simulink model "Sim_CVBT"  (R2022a)
settings: Solver=ode45  StartTime=0.0  StopTime=600  FixedStep=0.01  RelTol=1e-3  EnableMultiTasking=on
InitFcn:
  | initialize;
  | %graphics_init;
values from neighbouring files (symbols this model uses):
  a = 0.08    [initialize.m]
  b = 0.002*0    (= 0)    [initialize.m]
  Kdv = 0    [initialize.m]
  Kiv = 0    [initialize.m]
  Kpsi = 2    [initialize.m]
  Kpv = 0.2    [initialize.m]
  numVeh = 6    [initialize.m]
  P0 = zeros(40,1)    [initialize.m]
  P0tg = [-400 -400 0]    [initialize.m]
  psi0 = zeros(20,1)    [initialize.m]
  rho_d = [100 150 100 150 100 150 100 150 100 150]    [initialize.m]
  Vg = zeros(10,1)    [initialize.m]
  Vmax = 60    [initialize.m]
  Vmin = 10    [initialize.m]
  z0 = zeros(20,1)    [initialize.m]
libraries: slpidlib x6, simulink x2
(part 1 of 2)
settings Model: Creator=cichell2  LastModifiedBy=vcichella
settings SolverCC: AlgebraicLoopSolver=TrustRegion
settings DataIOCC: LimitDataPoints=on  SaveFormat=Array  SignalLoggingSaveFormat=ModelDataLogs  ReturnWorkspaceOutputs=off
settings OptimizationCC: ExpressionDepthLimit=2147483647  LifeSpan=inf
settings DebuggingCC: UnderspecifiedInitializationDetection=Classic  MergeDetectMultiDrivingBlocksExec=none  SolverPrmCheckMsg=warning  FcnCallInpInsideContextMsg=warning  UnconnectedInputMsg=warning  UnconnectedOutputMsg=warning  UnconnectedLineMsg=warning  StateNameClashWarn=warning  SFUnexpectedBacktrackingDiag=warning  SFNoUnconditionalDefaultTransitionDiag=warning  SFExecutionAtInitializationDiag=none  SFMachineParentedDataDiag=warning  ArithmeticOperatorsInVariantConditions=warning
settings HardwareCC: ProdBitPerPointer=32  ProdBitPerSizeT=32  ProdBitPerPtrDiffT=32  ProdLargestAtomicFloat=None  ProdIntDivRoundTo=Undefined  ProdEndianess=Unspecified  ProdWordSize=32  ProdHWDeviceType=32-bit Generic
settings ModelReferenceCC: PropagateSignalLabelsOutOfModel=off
settings SFSimCC: SimUseLocalCustomCode=off  CustomCodeUndefinedFunction=UseInterfaceOnly
settings RTWCC: RTWUseLocalCustomCode=off
settings CodeAppCC: StateflowObjectComments=on
settings GRTTargetCC: TargetLangStandard=C89/C90 (ANSI)  CombineOutputUpdateFcns=off  GRTInterface=on
settings ConfigComp: CovMetricSettings=dw  CovSaveCumulativeToWorkspaceVar=on  CovSaveSingleToWorkspaceVar=on  CovExternalEMLEnable=off

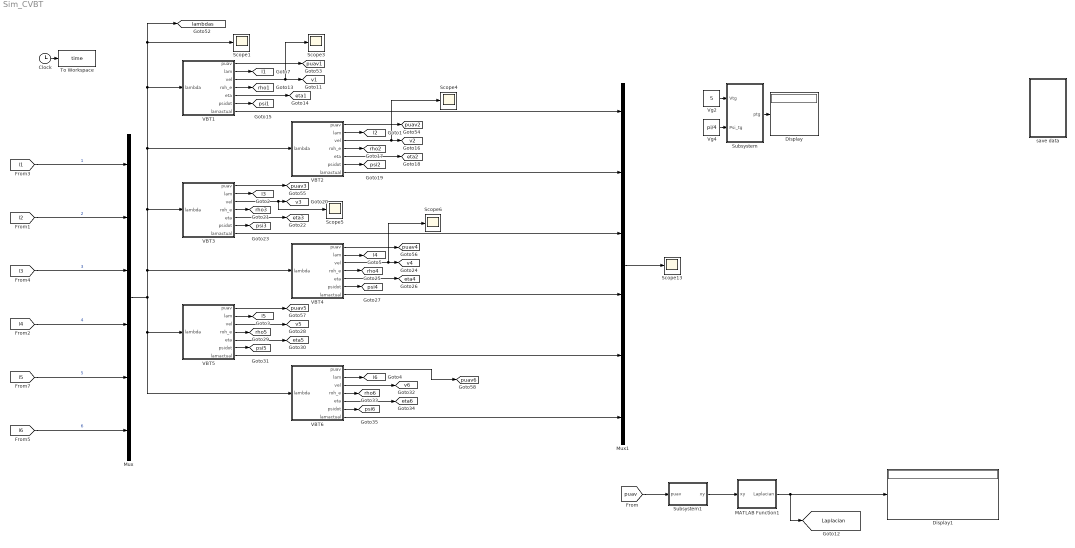
== system Sim_CVBT ==
  Clock : Clock
  Display : Display
  Display1 : Display
  MATLAB Function1 : MATLAB Function  TreatAsAtomicUnit=on
  Mux : Mux  Inputs=6
  Mux1 : Mux  Inputs=6
  Scope{1,3..6,13} (6 alike) : Scope
  Subsystem : Subsystem
  Subsystem1 : Subsystem
  To Workspace : ToWorkspace  VariableName=time  SampleTime=-1
  VBT1 : Subsystem  mask{UAV_no=1}
      mask prompts: UAV_no "UAV number"
  VBT2 : Subsystem  mask{UAV_no=2}
      mask prompts: UAV_no "UAV number"
  VBT3 : Subsystem  mask{UAV_no=3}
      mask prompts: UAV_no "UAV number"
  VBT4 : Subsystem  mask{UAV_no=4}
      mask prompts: UAV_no "UAV number"
  VBT5 : Subsystem  mask{UAV_no=5}
      mask prompts: UAV_no "UAV number"
  VBT6 : Subsystem  mask{UAV_no=6}
      mask prompts: UAV_no "UAV number"
  Vg2 : Constant  Value=5
  Vg4 : Constant  Value=pi/4
  save data : Subsystem
  tag scope: Laplacian=global, eta1=global, eta2=global, eta3=global, eta4=global, eta5=global, eta6=global, l1=global, l2=global, l3=global, l4=global, l5=global, l6=global, lambdas=global, psi1=global, psi2=global, psi3=global, psi4=global, psi5=global, psi6=global, puav1=global, puav2=global, puav3=global, puav4=global, puav5=global, puav6=global, rho1=global, rho2=global, rho3=global, rho4=global, rho5=global, rho6=global, v1=global, v2=global, v3=global, v4=global, v5=global, v6=global
  wires:
  Clock/1 -> To Workspace/1
  Vg2/1 -> Subsystem/1(Vtg)
  Vg4/1 -> Subsystem/2(Psi_tg)
  Subsystem/1(ptg) -> Display/1
  VBT1/2(lam) -> [l1]
  VBT2/2(lam) -> [l2]
  VBT3/2(lam) -> [l3]
  VBT5/2(lam) -> [l5]
  [l2] -> Mux/2  "2"
  [l1] -> Mux/1  "1"
  Mux/1 -> VBT5/1(lambda), VBT6/1(lambda), VBT3/1(lambda), [lambdas], Scope1/1, VBT1/1(lambda), VBT2/1(lambda), VBT4/1(lambda)
  [l4] -> Mux/4  "4"
  [l5] -> Mux/5  "5"
  [l6] -> Mux/6  "6"
  [l3] -> Mux/3  "3"
  VBT4/2(lam) -> [l4]
  VBT6/2(lam) -> [l6]
  VBT1/1(puav) -> [puav1]
  VBT2/1(puav) -> [puav2]
  VBT4/1(puav) -> [puav4]
  VBT5/1(puav) -> [puav5]
  VBT6/1(puav) -> [puav6]
  VBT1/3(vel) -> Scope3/1, [v1]
  VBT1/4(roh_e) -> [rho1]
  VBT1/5(eta) -> [eta1]
  VBT1/6(psidot) -> [psi1]
  VBT2/3(vel) -> Scope4/1, [v2]
  VBT2/5(eta) -> [eta2]
  VBT2/4(roh_e) -> [rho2]
  VBT2/6(psidot) -> [psi2]
  VBT3/3(vel) -> Scope5/1, [v3]
  VBT3/5(eta) -> [eta3]
  VBT3/4(roh_e) -> [rho3]
  VBT3/6(psidot) -> [psi3]
  VBT4/3(vel) -> Scope6/1, [v4]
  VBT4/5(eta) -> [eta4]
  VBT4/4(roh_e) -> [rho4]
  VBT4/6(psidot) -> [psi4]
  VBT5/3(vel) -> [v5]
  VBT5/5(eta) -> [eta5]
  VBT5/4(roh_e) -> [rho5]
  VBT5/6(psidot) -> [psi5]
  VBT6/3(vel) -> [v6]
  VBT6/5(eta) -> [eta6]
  VBT6/4(roh_e) -> [rho6]
  VBT6/6(psidot) -> [psi6]
  VBT3/1(puav) -> [puav3]
  [puav] -> Subsystem1/1(puav)
  MATLAB Function1/1(Laplacian) -> [Laplacian], Display1/1
  Subsystem1/1(xy) -> MATLAB Function1/1(xy)
  VBT1/7(lamactual) -> Mux1/1
  VBT2/7(lamactual) -> Mux1/2
  VBT3/7(lamactual) -> Mux1/3
  VBT4/7(lamactual) -> Mux1/4
  VBT5/7(lamactual) -> Mux1/5
  VBT6/7(lamactual) -> Mux1/6
  Mux1/1 -> Scope13/1

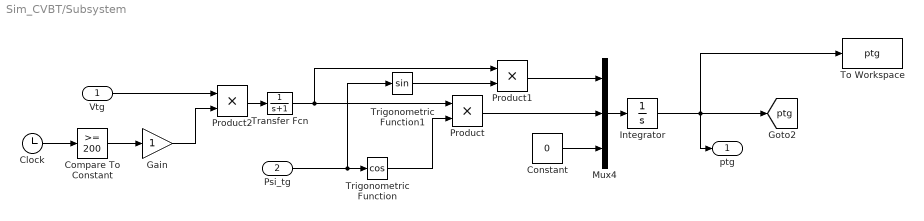
== system Sim_CVBT/Subsystem ==
  Vtg : Inport
  Psi_tg : Inport  Port=2
  Clock : Clock
  Compare To Constant : simulink/Logic and Bit Operations/Compare To Constant  relop=>=  const=200  OutDataTypeStr=boolean
  Constant : Constant  Value=0
  Gain : Gain
  Integrator : Integrator  InitialCondition=[P0tg(1) P0tg(2) P0tg(3)]  LimitOutput=on  UpperSaturationLimit=200  LowerSaturationLimit=-400
  Mux4 : Mux  Inputs=3
  Product : Product  RndMeth=Zero
  Product1 : Product  RndMeth=Zero
  Product2 : Product
  To Workspace : ToWorkspace  VariableName=ptg  SaveFormat=Timeseries  SampleTime=-1
  Transfer Fcn : TransferFcn  Denominator=[1 1]
  Trigonometric Function : Trigonometry  Operator=cos
  Trigonometric Function1 : Trigonometry
  ptg : Outport
  tag scope: ptg=global
  wires:
  Psi_tg/1 -> Trigonometric Function/1, Trigonometric Function1/1
  Integrator/1 -> To Workspace/1, ptg/1, [ptg]
  Mux4/1 -> Integrator/1
  Constant/1 -> Mux4/3
  Product/1 -> Mux4/2
  Trigonometric Function/1 -> Product/2
  Product1/1 -> Mux4/1
  Trigonometric Function1/1 -> Product1/2
  Clock/1 -> Compare To Constant/1
  Compare To Constant/1 -> Gain/1
  Product2/1 -> Transfer Fcn/1
  Vtg/1 -> Product2/1
  Gain/1 -> Product2/2
  Transfer Fcn/1 -> Product1/1, Product/1

== system Sim_CVBT/Subsystem1 ==
  puav : Inport
  Selector : Selector  InputPortWidth=18  IndexOptions=Index vector (dialog)  Indices=[1 2 4 5 7 8 10 11 13 14 16 17]  OutputSizes=1
  xy : Outport
  wires:
  puav/1 -> Selector/1
  Selector/1 -> xy/1

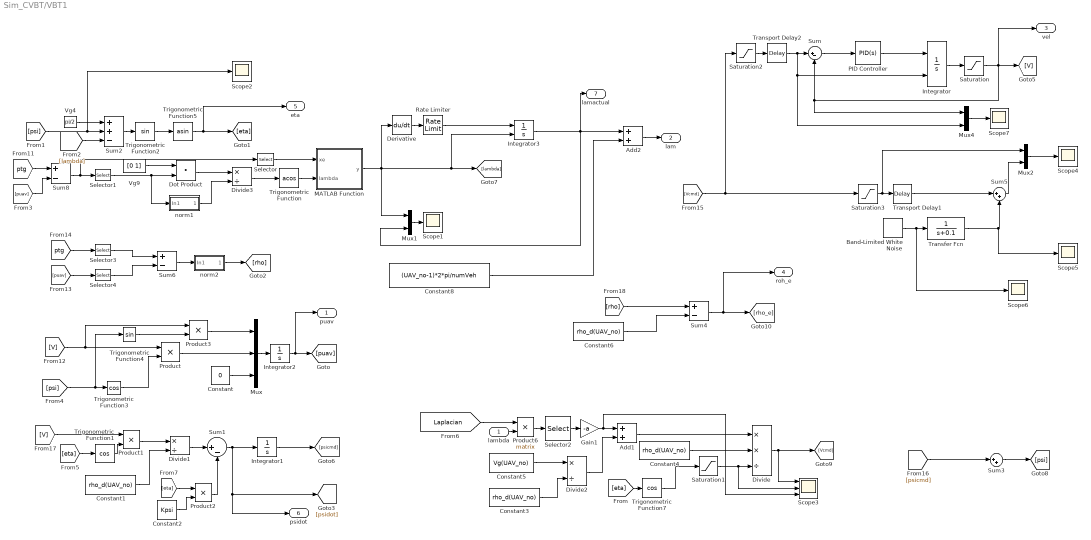
== system Sim_CVBT/VBT1 ==
  lambda : Inport
  Add1 : Sum
  Add2 : Sum
  Band-Limited White Noise : simulink/Sources/Band-Limited White Noise  Cov=[0.1]  Ts=0.1  seed=[23341]
  Constant : Constant  Value=0
  Constant{1,3..4,6} (4 alike) : Constant  Value=rho_d(UAV_no)
  Constant2 : Constant  Value=Kpsi
  Constant5 : Constant  Value=Vg(UAV_no)
  Constant8 : Constant  Value=(UAV_no-1)*2*pi/numVeh
  Derivative : Derivative
  Divide : Product  Inputs=**/
  Divide1 : Product  Inputs=*/
  Divide2 : Product  Inputs=*/
  Divide3 : Product  Inputs=*/
  Dot Product : DotProduct  OutDataTypeStr=Inherit: Inherit via internal rule
  Gain1 : Gain  Gain=-a
  Integrator : Integrator  InitialConditionSource=external
  Integrator1 : Integrator  InitialCondition=psi0(UAV_no)*pi/180
  Integrator2 : Integrator  InitialCondition=[P0(2*UAV_no-1) P0(2*UAV_no) z0(UAV_no)]
  Integrator3 : Integrator  InitialConditionSource=external
  MATLAB Function : MATLAB Function  TreatAsAtomicUnit=on
  Mux : Mux  Inputs=3
  Mux1 : Mux  Inputs=2
  Mux2 : Mux  Inputs=2
  Mux4 : Mux  Inputs=2
  PID Controller : slpidlib/PID Controller  Controller=PID  Form=Parallel  TimeDomain=Continuous-time  UseExternalTs=off  SampleTime=1  IntegratorMethod=Forward Euler  FilterMethod=Forward Euler  ControllerParametersSource=internal  P=Kpv  I=Kiv  UseKiTs=off  D=Kdv  N=100  UseFilter=on  TunerSelectOption=Transfer Function Based (PID Tuner App)  InitialConditionSource=internal  InitialConditionForIntegrator=0  InitialConditionForFilter=0  DifferentiatorICPrevScaledInput=0  ExternalReset=none  TrackingMode=off  Kt=1  LimitOutput=off  SatLimitsSource=internal  UpperSaturationLimit=inf  LowerSaturationLimit=-inf  LinearizeAsGain=on  AntiWindupMode=none  Kb=1  POutMin=[]  POutMax=[]  IOutMin=[]  IOutMax=[]  DOutMin=[]  DOutMax=[]  NOutMin=[]  NOutMax=[]  SumOutMin=[]  SumOutMax=[]  SaturationOutMin=[]  SaturationOutMax=[]  PParamMin=[]  PParamMax=[]  IParamMin=[]  IParamMax=[]  DParamMin=[]  DParamMax=[]  NParamMin=[]  NParamMax=[]  KbParamMin=[]  KbParamMax=[]  KtParamMin=[]  KtParamMax=[]  KbOutMin=[]  KbOutMax=[]  KtOutMin=[]  KtOutMax=[]  IntegratorOutMin=[]  IntegratorOutMax=[]  FilterOutMin=[]  FilterOutMax=[]  SumI1OutMin=[]  SumI1OutMax=[]  SumI2OutMin=[]  SumI2OutMax=[]  SumI3OutMin=[]  SumI3OutMax=[]  SumI4OutMin=[]  SumI4OutMax=[]  SumDOutMin=[]  SumDOutMax=[]  DifferentiatorOutMin=[]  DifferentiatorOutMax=[]  FilterDiffOutCoefMin=[]  FilterDiffOutCoefMax=[]  ReciprocalOutMin=[]  ReciprocalOutMax=[]  SumDenOutMin=[]  SumDenOutMax=[]  SumNumOutMin=[]  SumNumOutMax=[]  DivideOutMin=[]  DivideOutMax=[]  UdiffTsProdOutMin=[]  UdiffTsProdOutMax=[]  NTsProdOutMin=[]  NTsProdOutMax=[]  UintegralTsProdOutMin=[]  UintegralTsProdOutMax=[]  UngainTsProdOutMin=[]  UngainTsProdOutMax=[]  IntegratorContinuousStateAttributes=''  IntegratorStateMustResolveToSignalObject=off  IntegratorRTWStateStorageClass=Auto  FilterContinuousStateAttributes=''  FilterStateMustResolveToSignalObject=off  FilterRTWStateStorageClass=Auto  ParallelPVariant=InternalParameters  IdealPVariant=Disabled  IVariant=InternalParameters  DVariant=InternalParameters  IntegratorVariant=Continuous  SatVariant=Disabled  AWVariant=Passthrough  PCopyVariant=Disabled  TRVariant=Disabled  FdbkBlocksVariant=Forward  IdealPFdbkVariant=Disabled  SatFdbkVariant=Disabled  DerivativeFilterVariant=ContFilter  NVariant=InternalParameters  NCopyVariant=Disabled  FilterICVariant=InternalICsFilter  IntegratorICVariant=InternalICs  ExternalResetVariant=Disabled  TRSumVariant=Passthrough  SumFdbkVariant=Disabled  SumVariant=Sum_PID  TsampFilterVariant=InternalTs  TsampNgainVariant=Passthrough  TsampIntegralVariant=Passthrough  ExternalSaturationOutDataTypeStr=Inherit: Same as second input  aMode=0
  Product{,1..3} (4 alike) : Product  RndMeth=Zero
  Product6 : Product  Multiplication=Matrix(*)  RndMeth=Zero
  Rate Limiter : RateLimiter  RisingSlewLimit=100  FallingSlewLimit=-0.1  SampleTimeMode=inherited
  Saturation : Saturate  UpperLimit=Vmax  LowerLimit=Vmin
  Saturation1 : Saturate  UpperLimit=1  LowerLimit=0.8
  Saturation2 : Saturate  UpperLimit=Vmax  LowerLimit=Vmin
  Saturation3 : Saturate  UpperLimit=Vmax  LowerLimit=Vmin
  Scope{1..2,4..7} (6 alike) : Scope
  Scope3 : Scope  NumInputPorts=3
  Selector : Selector  InputPortWidth=3  IndexOptions=Index vector (dialog)  Indices=1  OutputSizes=1
  Selector1 : Selector  InputPortWidth=3  IndexOptions=Index vector (dialog)  Indices=[1 2]  OutputSizes=1
  Selector2 : Selector  InputPortWidth=6  IndexOptions=Index vector (dialog)  Indices=[UAV_no]  OutputSizes=1
  Selector3 : Selector  InputPortWidth=3  IndexOptions=Index vector (dialog)  Indices=[1 2]  OutputSizes=1
  Selector4 : Selector  InputPortWidth=3  IndexOptions=Index vector (dialog)  Indices=[1 2]  OutputSizes=1
  Sum : Sum  Inputs=|+-
  Sum1 : Sum  Inputs=|+-
  Sum2 : Sum  Inputs=++-
  Sum3 : Sum  Inputs=|++
  Sum4 : Sum  Inputs=+-
  Sum5 : Sum  Inputs=|++
  Sum6 : Sum  Inputs=+-
  Sum8 : Sum  Inputs=+-
  Transfer Fcn : TransferFcn  Denominator=[1 0.1]
  Transport Delay1 : TransportDelay  DelayTime=0.1
  Transport Delay2 : TransportDelay  DelayTime=0.1
  Trigonometric Function : Trigonometry  Operator=acos
  Trigonometric Function1 : Trigonometry  Operator=cos
  Trigonometric Function2 : Trigonometry
  Trigonometric Function3 : Trigonometry  Operator=cos
  Trigonometric Function4 : Trigonometry
  Trigonometric Function5 : Trigonometry  Operator=asin
  Trigonometric Function7 : Trigonometry  Operator=cos
  Vg4 : Constant  Value=pi/2
  Vg9 : Constant  Value=[0 1]
  norm1 : Subsystem
  norm2 : Subsystem
  puav : Outport
  lam : Outport  Port=2
  vel : Outport  Port=3
  roh_e : Outport  Port=4
  eta : Outport  Port=5
  psidot : Outport  Port=6
  lamactual : Outport  Port=7
  wires:
  Trigonometric Function1/1 -> Product1/2
  [eta] -> Trigonometric Function1/1
  Divide1/1 -> Sum1/1
  Product1/1 -> Divide1/1
  Constant1/1 -> Divide1/2
  [eta] -> Product2/1
  Product2/1 -> Sum1/2
  Constant2/1 -> Product2/2
  Sum1/1 -> Integrator1/1, psidot/1, [psidot]
  Sum6/1 -> norm2/1(In1)
  [puav] -> Selector4/1
  [ptg] -> Selector3/1
  Sum2/1 -> Trigonometric Function2/1
  Vg4/1 -> Sum2/1
  Sum8/1 -> Selector/1, Selector1/1
  [psi] -> Scope2/1, Sum2/2
  [lambda] -> Sum2/3
  Dot Product/1 -> Divide3/1
  norm1/1(Out1) -> Divide3/2
  [ptg] -> Sum8/1
  [puav] -> Sum8/2
  Integrator1/1 -> [psicmd]
  Selector/1 -> MATLAB Function/1(xe)
  Vg9/1 -> Dot Product/1
  Trigonometric Function2/1 -> Trigonometric Function5/1
  Trigonometric Function5/1 -> eta/1, [eta]
  [V] -> Product/1, Product3/1
  [psi] -> Trigonometric Function3/1, Trigonometric Function4/1
  Trigonometric Function3/1 -> Product/2
  Trigonometric Function4/1 -> Product3/2
  Product3/1 -> Mux/1
  Product/1 -> Mux/2
  Constant/1 -> Mux/3
  Mux/1 -> Integrator2/1
  Integrator2/1 -> puav/1, [puav]
  Selector1/1 -> Dot Product/2, norm1/1(In1)
  norm2/1(Out1) -> [rho]
  [V] -> Product1/1
  Mux1/1 -> Scope1/1
  [eta] -> Trigonometric Function7/1
  Add1/1 -> Divide/1
  Divide2/1 -> Add1/2
  Constant5/1 -> Divide2/1
  Constant3/1 -> Divide2/2
  Gain1/1 -> Scope3/3, Add1/1
  Trigonometric Function7/1 -> Saturation1/1
  Constant4/1 -> Divide/2
  Product6/1 -> Selector2/1
  [Laplacian] -> Product6/1
  lambda/1 -> Product6/2
  Selector2/1 -> Gain1/1
  Selector3/1 -> Sum6/1
  Selector4/1 -> Sum6/2
  Trigonometric Function/1 -> MATLAB Function/2(lambda)
  Divide3/1 -> Trigonometric Function/1
  MATLAB Function/1(y) -> Derivative/1, Mux1/1, Integrator3/2, [lambda]
  Derivative/1 -> Rate Limiter/1
  Integrator3/1 -> lamactual/1, Add2/1, Mux1/2
  Add2/1 -> lam/1
  Constant8/1 -> Add2/2
  Sum/1 -> PID Controller/1
  [psicmd] -> Sum3/1
  Sum3/1 -> [psi]
  [rho] -> Sum4/1
  Constant6/1 -> Sum4/2
  Sum4/1 -> roh_e/1, [rho_e]
  Saturation1/1 -> Scope3/2, Divide/3
  Saturation/1 -> [V], vel/1, Sum/2, Mux4/1
  Integrator/1 -> Saturation/1
  PID Controller/1 -> Integrator/1
  Mux4/1 -> Scope7/1
  Divide/1 -> Scope3/1, [Vcmd]
  Rate Limiter/1 -> Integrator3/1
  Saturation2/1 -> Transport Delay2/1
  [Vcmd] -> Saturation2/1, Saturation3/1
  Band-Limited White Noise/1 -> Scope6/1, Transfer Fcn/1
  Transfer Fcn/1 -> Scope5/1, Sum5/2
  Sum5/1 -> Mux2/2
  Mux2/1 -> Scope4/1
  Transport Delay1/1 -> Sum5/1
  Saturation3/1 -> Mux2/1, Transport Delay1/1
  Transport Delay2/1 -> Mux4/2, Integrator/2, Sum/1

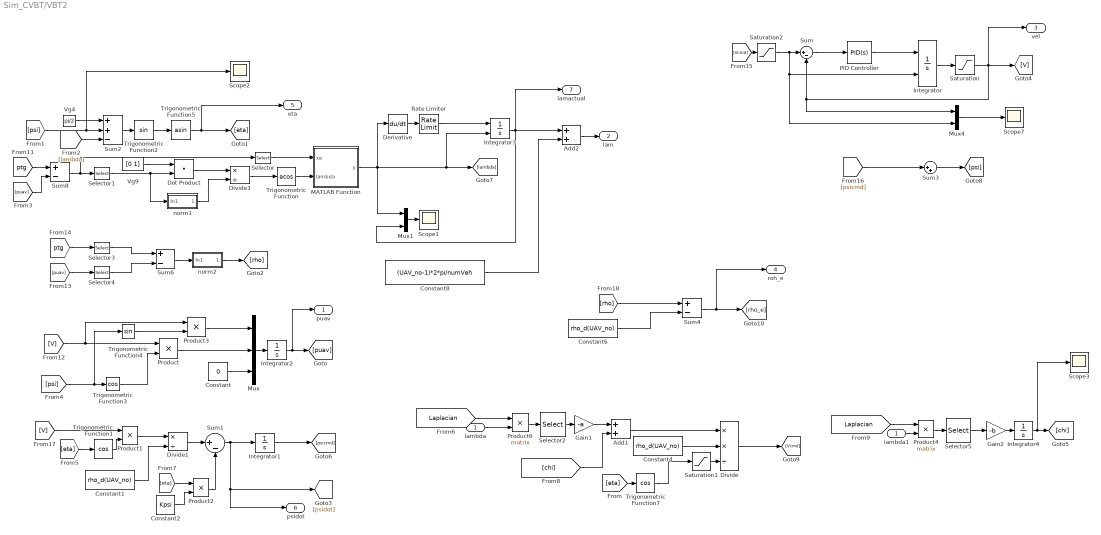
== system Sim_CVBT/VBT2 ==
  lambda : Inport
  Add1 : Sum
  Add2 : Sum
  Constant : Constant  Value=0
  Constant1 : Constant  Value=rho_d(UAV_no)
  Constant2 : Constant  Value=Kpsi
  Constant4 : Constant  Value=rho_d(UAV_no)
  Constant6 : Constant  Value=rho_d(UAV_no)
  Constant8 : Constant  Value=(UAV_no-1)*2*pi/numVeh
  Derivative : Derivative
  Divide : Product  Inputs=**/
  Divide1 : Product  Inputs=*/
  Divide3 : Product  Inputs=*/
  Dot Product : DotProduct  OutDataTypeStr=Inherit: Inherit via internal rule
  Gain1 : Gain  Gain=-a
  Gain2 : Gain  Gain=-b
  Integrator : Integrator  InitialConditionSource=external
  Integrator1 : Integrator  InitialCondition=psi0(UAV_no)*pi/180
  Integrator2 : Integrator  InitialCondition=[P0(2*UAV_no-1) P0(2*UAV_no) z0(UAV_no)]
  Integrator3 : Integrator  InitialConditionSource=external
  Integrator4 : Integrator  InitialCondition=Vg(UAV_no)/rho_d(UAV_no)
  MATLAB Function : MATLAB Function  TreatAsAtomicUnit=on
  Mux : Mux  Inputs=3
  Mux1 : Mux  Inputs=2
  Mux4 : Mux  Inputs=2
  PID Controller : slpidlib/PID Controller  Controller=PID  Form=Parallel  TimeDomain=Continuous-time  UseExternalTs=off  SampleTime=1  IntegratorMethod=Forward Euler  FilterMethod=Forward Euler  ControllerParametersSource=internal  P=Kpv  I=Kiv  UseKiTs=off  D=Kdv  N=100  UseFilter=on  TunerSelectOption=Transfer Function Based (PID Tuner App)  InitialConditionSource=internal  InitialConditionForIntegrator=0  InitialConditionForFilter=0  DifferentiatorICPrevScaledInput=0  ExternalReset=none  TrackingMode=off  Kt=1  LimitOutput=off  SatLimitsSource=internal  UpperSaturationLimit=inf  LowerSaturationLimit=-inf  LinearizeAsGain=on  AntiWindupMode=none  Kb=1  POutMin=[]  POutMax=[]  IOutMin=[]  IOutMax=[]  DOutMin=[]  DOutMax=[]  NOutMin=[]  NOutMax=[]  SumOutMin=[]  SumOutMax=[]  SaturationOutMin=[]  SaturationOutMax=[]  PParamMin=[]  PParamMax=[]  IParamMin=[]  IParamMax=[]  DParamMin=[]  DParamMax=[]  NParamMin=[]  NParamMax=[]  KbParamMin=[]  KbParamMax=[]  KtParamMin=[]  KtParamMax=[]  KbOutMin=[]  KbOutMax=[]  KtOutMin=[]  KtOutMax=[]  IntegratorOutMin=[]  IntegratorOutMax=[]  FilterOutMin=[]  FilterOutMax=[]  SumI1OutMin=[]  SumI1OutMax=[]  SumI2OutMin=[]  SumI2OutMax=[]  SumI3OutMin=[]  SumI3OutMax=[]  SumI4OutMin=[]  SumI4OutMax=[]  SumDOutMin=[]  SumDOutMax=[]  DifferentiatorOutMin=[]  DifferentiatorOutMax=[]  FilterDiffOutCoefMin=[]  FilterDiffOutCoefMax=[]  ReciprocalOutMin=[]  ReciprocalOutMax=[]  SumDenOutMin=[]  SumDenOutMax=[]  SumNumOutMin=[]  SumNumOutMax=[]  DivideOutMin=[]  DivideOutMax=[]  UdiffTsProdOutMin=[]  UdiffTsProdOutMax=[]  NTsProdOutMin=[]  NTsProdOutMax=[]  UintegralTsProdOutMin=[]  UintegralTsProdOutMax=[]  UngainTsProdOutMin=[]  UngainTsProdOutMax=[]  IntegratorContinuousStateAttributes=''  IntegratorStateMustResolveToSignalObject=off  IntegratorRTWStateStorageClass=Auto  FilterContinuousStateAttributes=''  FilterStateMustResolveToSignalObject=off  FilterRTWStateStorageClass=Auto  ParallelPVariant=InternalParameters  IdealPVariant=Disabled  IVariant=InternalParameters  DVariant=InternalParameters  IntegratorVariant=Continuous  SatVariant=Disabled  AWVariant=Passthrough  PCopyVariant=Disabled  TRVariant=Disabled  FdbkBlocksVariant=Forward  IdealPFdbkVariant=Disabled  SatFdbkVariant=Disabled  DerivativeFilterVariant=ContFilter  NVariant=InternalParameters  NCopyVariant=Disabled  FilterICVariant=InternalICsFilter  IntegratorICVariant=InternalICs  ExternalResetVariant=Disabled  TRSumVariant=Passthrough  SumFdbkVariant=Disabled  SumVariant=Sum_PID  TsampFilterVariant=InternalTs  TsampNgainVariant=Passthrough  TsampIntegralVariant=Passthrough  ExternalSaturationOutDataTypeStr=Inherit: Same as second input  aMode=0
  Product{,1..3} (4 alike) : Product  RndMeth=Zero
  Product4 : Product  Multiplication=Matrix(*)  RndMeth=Zero
  Product6 : Product  Multiplication=Matrix(*)  RndMeth=Zero
  Rate Limiter : RateLimiter  RisingSlewLimit=100  FallingSlewLimit=-0.1  SampleTimeMode=inherited
  Saturation : Saturate  UpperLimit=Vmax  LowerLimit=Vmin
  Saturation1 : Saturate  UpperLimit=1  LowerLimit=0.8
  Saturation2 : Saturate  UpperLimit=Vmax  LowerLimit=Vmin
  Scope{1..3,7} (4 alike) : Scope
  Selector : Selector  InputPortWidth=3  IndexOptions=Index vector (dialog)  Indices=1  OutputSizes=1
  Selector1 : Selector  InputPortWidth=3  IndexOptions=Index vector (dialog)  Indices=[1 2]  OutputSizes=1
  Selector2 : Selector  InputPortWidth=6  IndexOptions=Index vector (dialog)  Indices=[UAV_no]  OutputSizes=1
  Selector3 : Selector  InputPortWidth=3  IndexOptions=Index vector (dialog)  Indices=[1 2]  OutputSizes=1
  Selector4 : Selector  InputPortWidth=3  IndexOptions=Index vector (dialog)  Indices=[1 2]  OutputSizes=1
  Selector5 : Selector  InputPortWidth=6  IndexOptions=Index vector (dialog)  Indices=[UAV_no]  OutputSizes=1
  Sum : Sum  Inputs=|+-
  Sum1 : Sum  Inputs=|+-
  Sum2 : Sum  Inputs=++-
  Sum3 : Sum  Inputs=|++
  Sum4 : Sum  Inputs=+-
  Sum6 : Sum  Inputs=+-
  Sum8 : Sum  Inputs=+-
  Trigonometric Function : Trigonometry  Operator=acos
  Trigonometric Function1 : Trigonometry  Operator=cos
  Trigonometric Function2 : Trigonometry
  Trigonometric Function3 : Trigonometry  Operator=cos
  Trigonometric Function4 : Trigonometry
  Trigonometric Function5 : Trigonometry  Operator=asin
  Trigonometric Function7 : Trigonometry  Operator=cos
  Vg4 : Constant  Value=pi/2
  Vg9 : Constant  Value=[0 1]
  lambda1 : InportShadow
  norm1 : Subsystem
  norm2 : Subsystem
  puav : Outport
  lam : Outport  Port=2
  vel : Outport  Port=3
  roh_e : Outport  Port=4
  eta : Outport  Port=5
  psidot : Outport  Port=6
  lamactual : Outport  Port=7
  wires:
  Mux4/1 -> Scope7/1
  PID Controller/1 -> Integrator/1
  Integrator/1 -> Saturation/1
  Saturation/1 -> Mux4/1, Sum/2, [V], vel/1
  Saturation1/1 -> Divide/3
  Sum4/1 -> [rho_e], roh_e/1
  Constant6/1 -> Sum4/2
  [rho] -> Sum4/1
  Sum3/1 -> [psi]
  [psicmd] -> Sum3/1
  [Vcmd] -> Saturation2/1
  Sum/1 -> PID Controller/1
  Constant8/1 -> Add2/2
  Add2/1 -> lam/1
  Integrator3/1 -> lamactual/1, Mux1/2, Add2/1
  Derivative/1 -> Rate Limiter/1
  MATLAB Function/1(y) -> [lambda], Integrator3/2, Mux1/1, Derivative/1
  Divide3/1 -> Trigonometric Function/1
  Trigonometric Function/1 -> MATLAB Function/2(lambda)
  Selector4/1 -> Sum6/2
  Selector3/1 -> Sum6/1
  Selector2/1 -> Gain1/1
  Divide/1 -> [Vcmd]
  lambda/1 -> Product6/2
  [Laplacian] -> Product6/1
  Product6/1 -> Selector2/1
  Constant4/1 -> Divide/2
  Trigonometric Function7/1 -> Saturation1/1
  Gain1/1 -> Add1/1
  Add1/1 -> Divide/1
  [eta] -> Trigonometric Function7/1
  Mux1/1 -> Scope1/1
  [V] -> Product1/1
  norm2/1(Out1) -> [rho]
  Selector1/1 -> norm1/1(In1), Dot Product/2
  Integrator2/1 -> [puav], puav/1
  Mux/1 -> Integrator2/1
  Constant/1 -> Mux/3
  Product/1 -> Mux/2
  Product3/1 -> Mux/1
  Trigonometric Function4/1 -> Product3/2
  Trigonometric Function3/1 -> Product/2
  [psi] -> Trigonometric Function4/1, Trigonometric Function3/1
  [V] -> Product3/1, Product/1
  Trigonometric Function5/1 -> [eta], eta/1
  Trigonometric Function2/1 -> Trigonometric Function5/1
  Vg9/1 -> Dot Product/1
  Selector/1 -> MATLAB Function/1(xe)
  Integrator1/1 -> [psicmd]
  [puav] -> Sum8/2
  [ptg] -> Sum8/1
  norm1/1(Out1) -> Divide3/2
  Dot Product/1 -> Divide3/1
  [lambda] -> Sum2/3
  [psi] -> Sum2/2, Scope2/1
  Sum8/1 -> Selector1/1, Selector/1
  Vg4/1 -> Sum2/1
  Sum2/1 -> Trigonometric Function2/1
  [ptg] -> Selector3/1
  [puav] -> Selector4/1
  Sum6/1 -> norm2/1(In1)
  Sum1/1 -> [psidot], psidot/1, Integrator1/1
  Constant2/1 -> Product2/2
  Product2/1 -> Sum1/2
  [eta] -> Product2/1
  Constant1/1 -> Divide1/2
  Product1/1 -> Divide1/1
  Divide1/1 -> Sum1/1
  [eta] -> Trigonometric Function1/1
  Trigonometric Function1/1 -> Product1/2
  Rate Limiter/1 -> Integrator3/1
  [chi] -> Add1/2
  Selector5/1 -> Gain2/1
  lambda1/1 -> Product4/2
  [Laplacian] -> Product4/1
  Product4/1 -> Selector5/1
  Gain2/1 -> Integrator4/1
  Integrator4/1 -> Scope3/1, [chi]
  Saturation2/1 -> Sum/1, Integrator/2, Mux4/2

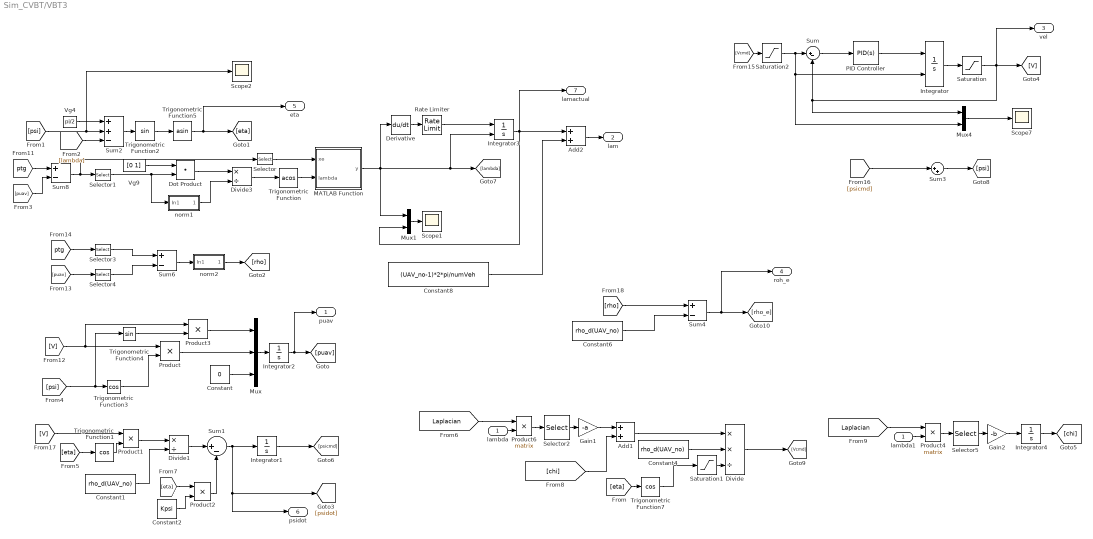
== system Sim_CVBT/VBT3 ==
  lambda : Inport
  Add1 : Sum
  Add2 : Sum
  Constant : Constant  Value=0
  Constant1 : Constant  Value=rho_d(UAV_no)
  Constant2 : Constant  Value=Kpsi
  Constant4 : Constant  Value=rho_d(UAV_no)
  Constant6 : Constant  Value=rho_d(UAV_no)
  Constant8 : Constant  Value=(UAV_no-1)*2*pi/numVeh
  Derivative : Derivative
  Divide : Product  Inputs=**/
  Divide1 : Product  Inputs=*/
  Divide3 : Product  Inputs=*/
  Dot Product : DotProduct  OutDataTypeStr=Inherit: Inherit via internal rule
  Gain1 : Gain  Gain=-a
  Gain2 : Gain  Gain=-b
  Integrator : Integrator  InitialConditionSource=external
  Integrator1 : Integrator  InitialCondition=psi0(UAV_no)*pi/180
  Integrator2 : Integrator  InitialCondition=[P0(2*UAV_no-1) P0(2*UAV_no) z0(UAV_no)]
  Integrator3 : Integrator  InitialConditionSource=external
  Integrator4 : Integrator  InitialCondition=Vg(UAV_no)/rho_d(UAV_no)
  MATLAB Function : MATLAB Function  TreatAsAtomicUnit=on
  Mux : Mux  Inputs=3
  Mux1 : Mux  Inputs=2
  Mux4 : Mux  Inputs=2
  PID Controller : slpidlib/PID Controller  Controller=PID  Form=Parallel  TimeDomain=Continuous-time  UseExternalTs=off  SampleTime=1  IntegratorMethod=Forward Euler  FilterMethod=Forward Euler  ControllerParametersSource=internal  P=Kpv  I=Kiv  UseKiTs=off  D=Kdv  N=100  UseFilter=on  TunerSelectOption=Transfer Function Based (PID Tuner App)  InitialConditionSource=internal  InitialConditionForIntegrator=0  InitialConditionForFilter=0  DifferentiatorICPrevScaledInput=0  ExternalReset=none  TrackingMode=off  Kt=1  LimitOutput=off  SatLimitsSource=internal  UpperSaturationLimit=inf  LowerSaturationLimit=-inf  LinearizeAsGain=on  AntiWindupMode=none  Kb=1  POutMin=[]  POutMax=[]  IOutMin=[]  IOutMax=[]  DOutMin=[]  DOutMax=[]  NOutMin=[]  NOutMax=[]  SumOutMin=[]  SumOutMax=[]  SaturationOutMin=[]  SaturationOutMax=[]  PParamMin=[]  PParamMax=[]  IParamMin=[]  IParamMax=[]  DParamMin=[]  DParamMax=[]  NParamMin=[]  NParamMax=[]  KbParamMin=[]  KbParamMax=[]  KtParamMin=[]  KtParamMax=[]  KbOutMin=[]  KbOutMax=[]  KtOutMin=[]  KtOutMax=[]  IntegratorOutMin=[]  IntegratorOutMax=[]  FilterOutMin=[]  FilterOutMax=[]  SumI1OutMin=[]  SumI1OutMax=[]  SumI2OutMin=[]  SumI2OutMax=[]  SumI3OutMin=[]  SumI3OutMax=[]  SumI4OutMin=[]  SumI4OutMax=[]  SumDOutMin=[]  SumDOutMax=[]  DifferentiatorOutMin=[]  DifferentiatorOutMax=[]  FilterDiffOutCoefMin=[]  FilterDiffOutCoefMax=[]  ReciprocalOutMin=[]  ReciprocalOutMax=[]  SumDenOutMin=[]  SumDenOutMax=[]  SumNumOutMin=[]  SumNumOutMax=[]  DivideOutMin=[]  DivideOutMax=[]  UdiffTsProdOutMin=[]  UdiffTsProdOutMax=[]  NTsProdOutMin=[]  NTsProdOutMax=[]  UintegralTsProdOutMin=[]  UintegralTsProdOutMax=[]  UngainTsProdOutMin=[]  UngainTsProdOutMax=[]  IntegratorContinuousStateAttributes=''  IntegratorStateMustResolveToSignalObject=off  IntegratorRTWStateStorageClass=Auto  FilterContinuousStateAttributes=''  FilterStateMustResolveToSignalObject=off  FilterRTWStateStorageClass=Auto  ParallelPVariant=InternalParameters  IdealPVariant=Disabled  IVariant=InternalParameters  DVariant=InternalParameters  IntegratorVariant=Continuous  SatVariant=Disabled  AWVariant=Passthrough  PCopyVariant=Disabled  TRVariant=Disabled  FdbkBlocksVariant=Forward  IdealPFdbkVariant=Disabled  SatFdbkVariant=Disabled  DerivativeFilterVariant=ContFilter  NVariant=InternalParameters  NCopyVariant=Disabled  FilterICVariant=InternalICsFilter  IntegratorICVariant=InternalICs  ExternalResetVariant=Disabled  TRSumVariant=Passthrough  SumFdbkVariant=Disabled  SumVariant=Sum_PID  TsampFilterVariant=InternalTs  TsampNgainVariant=Passthrough  TsampIntegralVariant=Passthrough  ExternalSaturationOutDataTypeStr=Inherit: Same as second input  aMode=0
  Product{,1..3} (4 alike) : Product  RndMeth=Zero
  Product4 : Product  Multiplication=Matrix(*)  RndMeth=Zero
  Product6 : Product  Multiplication=Matrix(*)  RndMeth=Zero
  Rate Limiter : RateLimiter  RisingSlewLimit=100  FallingSlewLimit=-0.1  SampleTimeMode=inherited
  Saturation : Saturate  UpperLimit=Vmax  LowerLimit=Vmin
  Saturation1 : Saturate  UpperLimit=1  LowerLimit=0.8
  Saturation2 : Saturate  UpperLimit=Vmax  LowerLimit=Vmin
  Scope1 : Scope
  Scope2 : Scope
  Scope7 : Scope
  Selector : Selector  InputPortWidth=3  IndexOptions=Index vector (dialog)  Indices=1  OutputSizes=1
  Selector1 : Selector  InputPortWidth=3  IndexOptions=Index vector (dialog)  Indices=[1 2]  OutputSizes=1
  Selector2 : Selector  InputPortWidth=6  IndexOptions=Index vector (dialog)  Indices=[UAV_no]  OutputSizes=1
  Selector3 : Selector  InputPortWidth=3  IndexOptions=Index vector (dialog)  Indices=[1 2]  OutputSizes=1
  Selector4 : Selector  InputPortWidth=3  IndexOptions=Index vector (dialog)  Indices=[1 2]  OutputSizes=1
  Selector5 : Selector  InputPortWidth=6  IndexOptions=Index vector (dialog)  Indices=[UAV_no]  OutputSizes=1
  Sum : Sum  Inputs=|+-
  Sum1 : Sum  Inputs=|+-
  Sum2 : Sum  Inputs=++-
  Sum3 : Sum  Inputs=|++
  Sum4 : Sum  Inputs=+-
  Sum6 : Sum  Inputs=+-
  Sum8 : Sum  Inputs=+-
  Trigonometric Function : Trigonometry  Operator=acos
  Trigonometric Function1 : Trigonometry  Operator=cos
  Trigonometric Function2 : Trigonometry
  Trigonometric Function3 : Trigonometry  Operator=cos
  Trigonometric Function4 : Trigonometry
  Trigonometric Function5 : Trigonometry  Operator=asin
  Trigonometric Function7 : Trigonometry  Operator=cos
  Vg4 : Constant  Value=pi/2
  Vg9 : Constant  Value=[0 1]
  lambda1 : InportShadow
  norm1 : Subsystem
  norm2 : Subsystem
  puav : Outport
  lam : Outport  Port=2
  vel : Outport  Port=3
  roh_e : Outport  Port=4
  eta : Outport  Port=5
  psidot : Outport  Port=6
  lamactual : Outport  Port=7
  wires:
  Integrator4/1 -> [chi]
  Gain2/1 -> Integrator4/1
  Product4/1 -> Selector5/1
  [Laplacian] -> Product4/1
  lambda1/1 -> Product4/2
  Selector5/1 -> Gain2/1
  [chi] -> Add1/2
  Rate Limiter/1 -> Integrator3/1
  Trigonometric Function1/1 -> Product1/2
  [eta] -> Trigonometric Function1/1
  Divide1/1 -> Sum1/1
  Product1/1 -> Divide1/1
  Constant1/1 -> Divide1/2
  [eta] -> Product2/1
  Product2/1 -> Sum1/2
  Constant2/1 -> Product2/2
  Sum1/1 -> Integrator1/1, psidot/1, [psidot]
  Sum6/1 -> norm2/1(In1)
  [puav] -> Selector4/1
  [ptg] -> Selector3/1
  Sum2/1 -> Trigonometric Function2/1
  Vg4/1 -> Sum2/1
  Sum8/1 -> Selector/1, Selector1/1
  [psi] -> Scope2/1, Sum2/2
  [lambda] -> Sum2/3
  Dot Product/1 -> Divide3/1
  norm1/1(Out1) -> Divide3/2
  [ptg] -> Sum8/1
  [puav] -> Sum8/2
  Integrator1/1 -> [psicmd]
  Selector/1 -> MATLAB Function/1(xe)
  Vg9/1 -> Dot Product/1
  Trigonometric Function2/1 -> Trigonometric Function5/1
  Trigonometric Function5/1 -> eta/1, [eta]
  [V] -> Product/1, Product3/1
  [psi] -> Trigonometric Function3/1, Trigonometric Function4/1
  Trigonometric Function3/1 -> Product/2
  Trigonometric Function4/1 -> Product3/2
  Product3/1 -> Mux/1
  Product/1 -> Mux/2
  Constant/1 -> Mux/3
  Mux/1 -> Integrator2/1
  Integrator2/1 -> puav/1, [puav]
  Selector1/1 -> Dot Product/2, norm1/1(In1)
  norm2/1(Out1) -> [rho]
  [V] -> Product1/1
  Mux1/1 -> Scope1/1
  [eta] -> Trigonometric Function7/1
  Add1/1 -> Divide/1
  Gain1/1 -> Add1/1
  Trigonometric Function7/1 -> Saturation1/1
  Constant4/1 -> Divide/2
  Product6/1 -> Selector2/1
  [Laplacian] -> Product6/1
  lambda/1 -> Product6/2
  Divide/1 -> [Vcmd]
  Selector2/1 -> Gain1/1
  Selector3/1 -> Sum6/1
  Selector4/1 -> Sum6/2
  Trigonometric Function/1 -> MATLAB Function/2(lambda)
  Divide3/1 -> Trigonometric Function/1
  MATLAB Function/1(y) -> Derivative/1, Mux1/1, Integrator3/2, [lambda]
  Derivative/1 -> Rate Limiter/1
  Integrator3/1 -> Add2/1, Mux1/2, lamactual/1
  Add2/1 -> lam/1
  Constant8/1 -> Add2/2
  Sum/1 -> PID Controller/1
  [Vcmd] -> Saturation2/1
  [psicmd] -> Sum3/1
  Sum3/1 -> [psi]
  [rho] -> Sum4/1
  Constant6/1 -> Sum4/2
  Sum4/1 -> roh_e/1, [rho_e]
  Saturation1/1 -> Divide/3
  Saturation/1 -> vel/1, [V], Sum/2, Mux4/1
  Integrator/1 -> Saturation/1
  PID Controller/1 -> Integrator/1
  Mux4/1 -> Scope7/1
  Saturation2/1 -> Mux4/2, Integrator/2, Sum/1

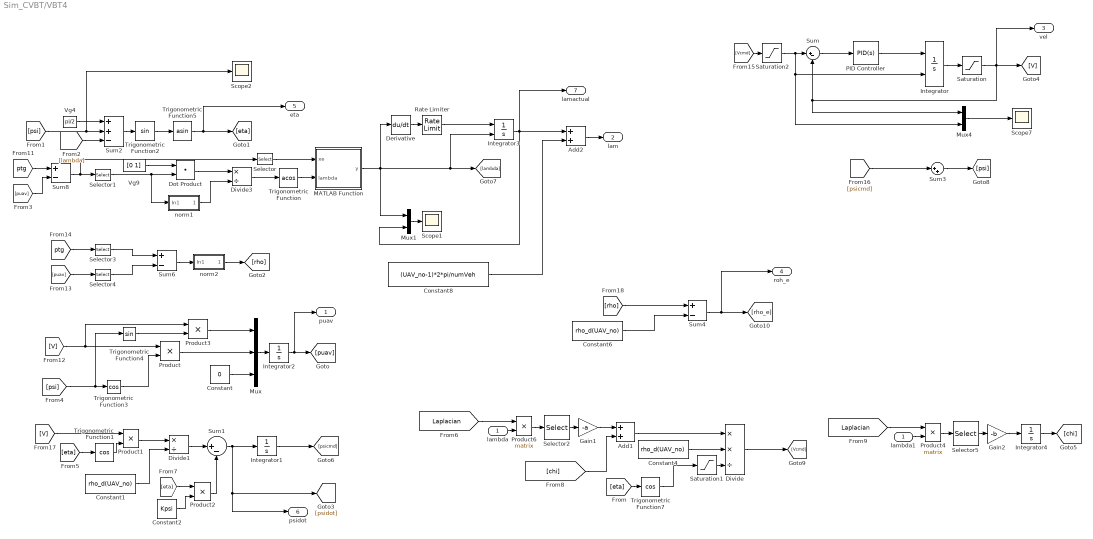
== system Sim_CVBT/VBT4 ==
  lambda : Inport
  Add1 : Sum
  Add2 : Sum
  Constant : Constant  Value=0
  Constant1 : Constant  Value=rho_d(UAV_no)
  Constant2 : Constant  Value=Kpsi
  Constant4 : Constant  Value=rho_d(UAV_no)
  Constant6 : Constant  Value=rho_d(UAV_no)
  Constant8 : Constant  Value=(UAV_no-1)*2*pi/numVeh
  Derivative : Derivative
  Divide : Product  Inputs=**/
  Divide1 : Product  Inputs=*/
  Divide3 : Product  Inputs=*/
  Dot Product : DotProduct  OutDataTypeStr=Inherit: Inherit via internal rule
  Gain1 : Gain  Gain=-a
  Gain2 : Gain  Gain=-b
  Integrator : Integrator  InitialConditionSource=external
  Integrator1 : Integrator  InitialCondition=psi0(UAV_no)*pi/180
  Integrator2 : Integrator  InitialCondition=[P0(2*UAV_no-1) P0(2*UAV_no) z0(UAV_no)]
  Integrator3 : Integrator  InitialConditionSource=external
  Integrator4 : Integrator  InitialCondition=Vg(UAV_no)/rho_d(UAV_no)
  MATLAB Function : MATLAB Function  TreatAsAtomicUnit=on
  Mux : Mux  Inputs=3
  Mux1 : Mux  Inputs=2
  Mux4 : Mux  Inputs=2
  PID Controller : slpidlib/PID Controller  Controller=PID  Form=Parallel  TimeDomain=Continuous-time  UseExternalTs=off  SampleTime=1  IntegratorMethod=Forward Euler  FilterMethod=Forward Euler  ControllerParametersSource=internal  P=Kpv  I=Kiv  UseKiTs=off  D=Kdv  N=100  UseFilter=on  TunerSelectOption=Transfer Function Based (PID Tuner App)  InitialConditionSource=internal  InitialConditionForIntegrator=0  InitialConditionForFilter=0  DifferentiatorICPrevScaledInput=0  ExternalReset=none  TrackingMode=off  Kt=1  LimitOutput=off  SatLimitsSource=internal  UpperSaturationLimit=inf  LowerSaturationLimit=-inf  LinearizeAsGain=on  AntiWindupMode=none  Kb=1  POutMin=[]  POutMax=[]  IOutMin=[]  IOutMax=[]  DOutMin=[]  DOutMax=[]  NOutMin=[]  NOutMax=[]  SumOutMin=[]  SumOutMax=[]  SaturationOutMin=[]  SaturationOutMax=[]  PParamMin=[]  PParamMax=[]  IParamMin=[]  IParamMax=[]  DParamMin=[]  DParamMax=[]  NParamMin=[]  NParamMax=[]  KbParamMin=[]  KbParamMax=[]  KtParamMin=[]  KtParamMax=[]  KbOutMin=[]  KbOutMax=[]  KtOutMin=[]  KtOutMax=[]  IntegratorOutMin=[]  IntegratorOutMax=[]  FilterOutMin=[]  FilterOutMax=[]  SumI1OutMin=[]  SumI1OutMax=[]  SumI2OutMin=[]  SumI2OutMax=[]  SumI3OutMin=[]  SumI3OutMax=[]  SumI4OutMin=[]  SumI4OutMax=[]  SumDOutMin=[]  SumDOutMax=[]  DifferentiatorOutMin=[]  DifferentiatorOutMax=[]  FilterDiffOutCoefMin=[]  FilterDiffOutCoefMax=[]  ReciprocalOutMin=[]  ReciprocalOutMax=[]  SumDenOutMin=[]  SumDenOutMax=[]  SumNumOutMin=[]  SumNumOutMax=[]  DivideOutMin=[]  DivideOutMax=[]  UdiffTsProdOutMin=[]  UdiffTsProdOutMax=[]  NTsProdOutMin=[]  NTsProdOutMax=[]  UintegralTsProdOutMin=[]  UintegralTsProdOutMax=[]  UngainTsProdOutMin=[]  UngainTsProdOutMax=[]  IntegratorContinuousStateAttributes=''  IntegratorStateMustResolveToSignalObject=off  IntegratorRTWStateStorageClass=Auto  FilterContinuousStateAttributes=''  FilterStateMustResolveToSignalObject=off  FilterRTWStateStorageClass=Auto  ParallelPVariant=InternalParameters  IdealPVariant=Disabled  IVariant=InternalParameters  DVariant=InternalParameters  IntegratorVariant=Continuous  SatVariant=Disabled  AWVariant=Passthrough  PCopyVariant=Disabled  TRVariant=Disabled  FdbkBlocksVariant=Forward  IdealPFdbkVariant=Disabled  SatFdbkVariant=Disabled  DerivativeFilterVariant=ContFilter  NVariant=InternalParameters  NCopyVariant=Disabled  FilterICVariant=InternalICsFilter  IntegratorICVariant=InternalICs  ExternalResetVariant=Disabled  TRSumVariant=Passthrough  SumFdbkVariant=Disabled  SumVariant=Sum_PID  TsampFilterVariant=InternalTs  TsampNgainVariant=Passthrough  TsampIntegralVariant=Passthrough  ExternalSaturationOutDataTypeStr=Inherit: Same as second input  aMode=0
  Product{,1..3} (4 alike) : Product  RndMeth=Zero
  Product4 : Product  Multiplication=Matrix(*)  RndMeth=Zero
  Product6 : Product  Multiplication=Matrix(*)  RndMeth=Zero
  Rate Limiter : RateLimiter  RisingSlewLimit=100  FallingSlewLimit=-0.1  SampleTimeMode=inherited
  Saturation : Saturate  UpperLimit=Vmax  LowerLimit=Vmin
  Saturation1 : Saturate  UpperLimit=1  LowerLimit=0.8
  Saturation2 : Saturate  UpperLimit=Vmax  LowerLimit=Vmin
  Scope1 : Scope
  Scope2 : Scope
  Scope7 : Scope
  Selector : Selector  InputPortWidth=3  IndexOptions=Index vector (dialog)  Indices=1  OutputSizes=1
  Selector1 : Selector  InputPortWidth=3  IndexOptions=Index vector (dialog)  Indices=[1 2]  OutputSizes=1
  Selector2 : Selector  InputPortWidth=6  IndexOptions=Index vector (dialog)  Indices=[UAV_no]  OutputSizes=1
  Selector3 : Selector  InputPortWidth=3  IndexOptions=Index vector (dialog)  Indices=[1 2]  OutputSizes=1
  Selector4 : Selector  InputPortWidth=3  IndexOptions=Index vector (dialog)  Indices=[1 2]  OutputSizes=1
  Selector5 : Selector  InputPortWidth=6  IndexOptions=Index vector (dialog)  Indices=[UAV_no]  OutputSizes=1
  Sum : Sum  Inputs=|+-
  Sum1 : Sum  Inputs=|+-
  Sum2 : Sum  Inputs=++-
  Sum3 : Sum  Inputs=|++
  Sum4 : Sum  Inputs=+-
  Sum6 : Sum  Inputs=+-
  Sum8 : Sum  Inputs=+-
  Trigonometric Function : Trigonometry  Operator=acos
  Trigonometric Function1 : Trigonometry  Operator=cos
  Trigonometric Function2 : Trigonometry
  Trigonometric Function3 : Trigonometry  Operator=cos
  Trigonometric Function4 : Trigonometry
  Trigonometric Function5 : Trigonometry  Operator=asin
  Trigonometric Function7 : Trigonometry  Operator=cos
  Vg4 : Constant  Value=pi/2
  Vg9 : Constant  Value=[0 1]
  lambda1 : InportShadow
  norm1 : Subsystem
  norm2 : Subsystem
  puav : Outport
  lam : Outport  Port=2
  vel : Outport  Port=3
  roh_e : Outport  Port=4
  eta : Outport  Port=5
  psidot : Outport  Port=6
  lamactual : Outport  Port=7
  wires:
  Mux4/1 -> Scope7/1
  PID Controller/1 -> Integrator/1
  Integrator/1 -> Saturation/1
  Saturation/1 -> Mux4/1, Sum/2, [V], vel/1
  Saturation1/1 -> Divide/3
  Sum4/1 -> [rho_e], roh_e/1
  Constant6/1 -> Sum4/2
  [rho] -> Sum4/1
  Sum3/1 -> [psi]
  [psicmd] -> Sum3/1
  [Vcmd] -> Saturation2/1
  Sum/1 -> PID Controller/1
  Constant8/1 -> Add2/2
  Add2/1 -> lam/1
  Integrator3/1 -> lamactual/1, Mux1/2, Add2/1
  Derivative/1 -> Rate Limiter/1
  MATLAB Function/1(y) -> [lambda], Integrator3/2, Mux1/1, Derivative/1
  Divide3/1 -> Trigonometric Function/1
  Trigonometric Function/1 -> MATLAB Function/2(lambda)
  Selector4/1 -> Sum6/2
  Selector3/1 -> Sum6/1
  Selector2/1 -> Gain1/1
  Divide/1 -> [Vcmd]
  lambda/1 -> Product6/2
  [Laplacian] -> Product6/1
  Product6/1 -> Selector2/1
  Constant4/1 -> Divide/2
  Trigonometric Function7/1 -> Saturation1/1
  Gain1/1 -> Add1/1
  Add1/1 -> Divide/1
  [eta] -> Trigonometric Function7/1
  Mux1/1 -> Scope1/1
  [V] -> Product1/1
  norm2/1(Out1) -> [rho]
  Selector1/1 -> norm1/1(In1), Dot Product/2
  Integrator2/1 -> [puav], puav/1
  Mux/1 -> Integrator2/1
  Constant/1 -> Mux/3
  Product/1 -> Mux/2
  Product3/1 -> Mux/1
  Trigonometric Function4/1 -> Product3/2
  Trigonometric Function3/1 -> Product/2
  [psi] -> Trigonometric Function4/1, Trigonometric Function3/1
  [V] -> Product3/1, Product/1
  Trigonometric Function5/1 -> [eta], eta/1
  Trigonometric Function2/1 -> Trigonometric Function5/1
  Vg9/1 -> Dot Product/1
  Selector/1 -> MATLAB Function/1(xe)
  Integrator1/1 -> [psicmd]
  [puav] -> Sum8/2
  [ptg] -> Sum8/1
  norm1/1(Out1) -> Divide3/2
  Dot Product/1 -> Divide3/1
  [lambda] -> Sum2/3
  [psi] -> Sum2/2, Scope2/1
  Sum8/1 -> Selector1/1, Selector/1
  Vg4/1 -> Sum2/1
  Sum2/1 -> Trigonometric Function2/1
  [ptg] -> Selector3/1
  [puav] -> Selector4/1
  Sum6/1 -> norm2/1(In1)
  Sum1/1 -> [psidot], psidot/1, Integrator1/1
  Constant2/1 -> Product2/2
  Product2/1 -> Sum1/2
  [eta] -> Product2/1
  Constant1/1 -> Divide1/2
  Product1/1 -> Divide1/1
  Divide1/1 -> Sum1/1
  [eta] -> Trigonometric Function1/1
  Trigonometric Function1/1 -> Product1/2
  Rate Limiter/1 -> Integrator3/1
  [chi] -> Add1/2
  Selector5/1 -> Gain2/1
  lambda1/1 -> Product4/2
  [Laplacian] -> Product4/1
  Product4/1 -> Selector5/1
  Gain2/1 -> Integrator4/1
  Integrator4/1 -> [chi]
  Saturation2/1 -> Sum/1, Integrator/2, Mux4/2

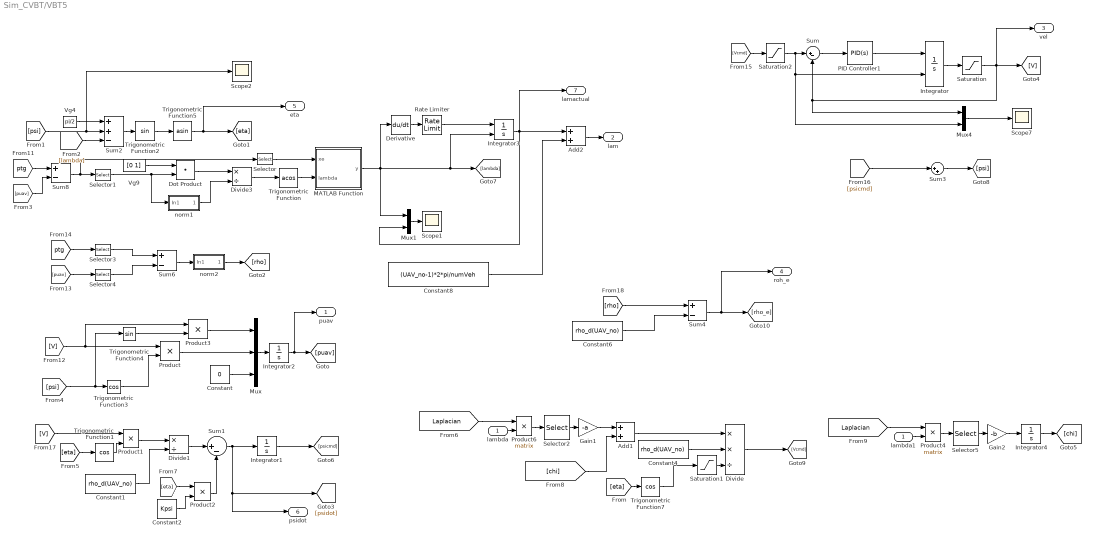
== system Sim_CVBT/VBT5 ==
  lambda : Inport
  Add1 : Sum
  Add2 : Sum
  Constant : Constant  Value=0
  Constant1 : Constant  Value=rho_d(UAV_no)
  Constant2 : Constant  Value=Kpsi
  Constant4 : Constant  Value=rho_d(UAV_no)
  Constant6 : Constant  Value=rho_d(UAV_no)
  Constant8 : Constant  Value=(UAV_no-1)*2*pi/numVeh
  Derivative : Derivative
  Divide : Product  Inputs=**/
  Divide1 : Product  Inputs=*/
  Divide3 : Product  Inputs=*/
  Dot Product : DotProduct  OutDataTypeStr=Inherit: Inherit via internal rule
  Gain1 : Gain  Gain=-a
  Gain2 : Gain  Gain=-b
  Integrator : Integrator  InitialConditionSource=external
  Integrator1 : Integrator  InitialCondition=psi0(UAV_no)*pi/180
  Integrator2 : Integrator  InitialCondition=[P0(2*UAV_no-1) P0(2*UAV_no) z0(UAV_no)]
  Integrator3 : Integrator  InitialConditionSource=external
  Integrator4 : Integrator  InitialCondition=Vg(UAV_no)/rho_d(UAV_no)
  MATLAB Function : MATLAB Function  TreatAsAtomicUnit=on
  Mux : Mux  Inputs=3
  Mux1 : Mux  Inputs=2
  Mux4 : Mux  Inputs=2
  PID Controller1 : slpidlib/PID Controller  Controller=PID  Form=Parallel  TimeDomain=Continuous-time  UseExternalTs=off  SampleTime=1  IntegratorMethod=Forward Euler  FilterMethod=Forward Euler  ControllerParametersSource=internal  P=Kpv  I=Kiv  UseKiTs=off  D=Kdv  N=100  UseFilter=on  TunerSelectOption=Transfer Function Based (PID Tuner App)  InitialConditionSource=internal  InitialConditionForIntegrator=0  InitialConditionForFilter=0  DifferentiatorICPrevScaledInput=0  ExternalReset=none  TrackingMode=off  Kt=1  LimitOutput=off  SatLimitsSource=internal  UpperSaturationLimit=inf  LowerSaturationLimit=-inf  LinearizeAsGain=on  AntiWindupMode=none  Kb=1  POutMin=[]  POutMax=[]  IOutMin=[]  IOutMax=[]  DOutMin=[]  DOutMax=[]  NOutMin=[]  NOutMax=[]  SumOutMin=[]  SumOutMax=[]  SaturationOutMin=[]  SaturationOutMax=[]  PParamMin=[]  PParamMax=[]  IParamMin=[]  IParamMax=[]  DParamMin=[]  DParamMax=[]  NParamMin=[]  NParamMax=[]  KbParamMin=[]  KbParamMax=[]  KtParamMin=[]  KtParamMax=[]  KbOutMin=[]  KbOutMax=[]  KtOutMin=[]  KtOutMax=[]  IntegratorOutMin=[]  IntegratorOutMax=[]  FilterOutMin=[]  FilterOutMax=[]  SumI1OutMin=[]  SumI1OutMax=[]  SumI2OutMin=[]  SumI2OutMax=[]  SumI3OutMin=[]  SumI3OutMax=[]  SumI4OutMin=[]  SumI4OutMax=[]  SumDOutMin=[]  SumDOutMax=[]  DifferentiatorOutMin=[]  DifferentiatorOutMax=[]  FilterDiffOutCoefMin=[]  FilterDiffOutCoefMax=[]  ReciprocalOutMin=[]  ReciprocalOutMax=[]  SumDenOutMin=[]  SumDenOutMax=[]  SumNumOutMin=[]  SumNumOutMax=[]  DivideOutMin=[]  DivideOutMax=[]  UdiffTsProdOutMin=[]  UdiffTsProdOutMax=[]  NTsProdOutMin=[]  NTsProdOutMax=[]  UintegralTsProdOutMin=[]  UintegralTsProdOutMax=[]  UngainTsProdOutMin=[]  UngainTsProdOutMax=[]  IntegratorContinuousStateAttributes=''  IntegratorStateMustResolveToSignalObject=off  IntegratorRTWStateStorageClass=Auto  FilterContinuousStateAttributes=''  FilterStateMustResolveToSignalObject=off  FilterRTWStateStorageClass=Auto  ParallelPVariant=InternalParameters  IdealPVariant=Disabled  IVariant=InternalParameters  DVariant=InternalParameters  IntegratorVariant=Continuous  SatVariant=Disabled  AWVariant=Passthrough  PCopyVariant=Disabled  TRVariant=Disabled  FdbkBlocksVariant=Forward  IdealPFdbkVariant=Disabled  SatFdbkVariant=Disabled  DerivativeFilterVariant=ContFilter  NVariant=InternalParameters  NCopyVariant=Disabled  FilterICVariant=InternalICsFilter  IntegratorICVariant=InternalICs  ExternalResetVariant=Disabled  TRSumVariant=Passthrough  SumFdbkVariant=Disabled  SumVariant=Sum_PID  TsampFilterVariant=InternalTs  TsampNgainVariant=Passthrough  TsampIntegralVariant=Passthrough  ExternalSaturationOutDataTypeStr=Inherit: Same as second input  aMode=0
  Product{,1..3} (4 alike) : Product  RndMeth=Zero
  Product4 : Product  Multiplication=Matrix(*)  RndMeth=Zero
  Product6 : Product  Multiplication=Matrix(*)  RndMeth=Zero
  Rate Limiter : RateLimiter  RisingSlewLimit=100  FallingSlewLimit=-0.1  SampleTimeMode=inherited
  Saturation : Saturate  UpperLimit=Vmax  LowerLimit=Vmin
  Saturation1 : Saturate  UpperLimit=1  LowerLimit=0.8
  Saturation2 : Saturate  UpperLimit=Vmax  LowerLimit=Vmin
  Scope1 : Scope
  Scope2 : Scope
  Scope7 : Scope
  Selector : Selector  InputPortWidth=3  IndexOptions=Index vector (dialog)  Indices=1  OutputSizes=1
  Selector1 : Selector  InputPortWidth=3  IndexOptions=Index vector (dialog)  Indices=[1 2]  OutputSizes=1
  Selector2 : Selector  InputPortWidth=6  IndexOptions=Index vector (dialog)  Indices=[UAV_no]  OutputSizes=1
  Selector3 : Selector  InputPortWidth=3  IndexOptions=Index vector (dialog)  Indices=[1 2]  OutputSizes=1
  Selector4 : Selector  InputPortWidth=3  IndexOptions=Index vector (dialog)  Indices=[1 2]  OutputSizes=1
  Selector5 : Selector  InputPortWidth=6  IndexOptions=Index vector (dialog)  Indices=[UAV_no]  OutputSizes=1
  Sum : Sum  Inputs=|+-
  Sum1 : Sum  Inputs=|+-
  Sum2 : Sum  Inputs=++-
  Sum3 : Sum  Inputs=|++
  Sum4 : Sum  Inputs=+-
  Sum6 : Sum  Inputs=+-
  Sum8 : Sum  Inputs=+-
  Trigonometric Function : Trigonometry  Operator=acos
  Trigonometric Function1 : Trigonometry  Operator=cos
  Trigonometric Function2 : Trigonometry
  Trigonometric Function3 : Trigonometry  Operator=cos
  Trigonometric Function4 : Trigonometry
  Trigonometric Function5 : Trigonometry  Operator=asin
  Trigonometric Function7 : Trigonometry  Operator=cos
  Vg4 : Constant  Value=pi/2
  Vg9 : Constant  Value=[0 1]
  lambda1 : InportShadow
  norm1 : Subsystem
  norm2 : Subsystem
  puav : Outport
  lam : Outport  Port=2
  vel : Outport  Port=3
  roh_e : Outport  Port=4
  eta : Outport  Port=5
  psidot : Outport  Port=6
  lamactual : Outport  Port=7
  wires:
  Integrator4/1 -> [chi]
  Gain2/1 -> Integrator4/1
  Product4/1 -> Selector5/1
  [Laplacian] -> Product4/1
  lambda1/1 -> Product4/2
  Selector5/1 -> Gain2/1
  [chi] -> Add1/2
  Rate Limiter/1 -> Integrator3/1
  Trigonometric Function1/1 -> Product1/2
  [eta] -> Trigonometric Function1/1
  Divide1/1 -> Sum1/1
  Product1/1 -> Divide1/1
  Constant1/1 -> Divide1/2
  [eta] -> Product2/1
  Product2/1 -> Sum1/2
  Constant2/1 -> Product2/2
  Sum1/1 -> Integrator1/1, psidot/1, [psidot]
  Sum6/1 -> norm2/1(In1)
  [puav] -> Selector4/1
  [ptg] -> Selector3/1
  Sum2/1 -> Trigonometric Function2/1
  Vg4/1 -> Sum2/1
  Sum8/1 -> Selector/1, Selector1/1
  [psi] -> Scope2/1, Sum2/2
  [lambda] -> Sum2/3
  Dot Product/1 -> Divide3/1
  norm1/1(Out1) -> Divide3/2
  [ptg] -> Sum8/1
  [puav] -> Sum8/2
  Integrator1/1 -> [psicmd]
  Selector/1 -> MATLAB Function/1(xe)
  Vg9/1 -> Dot Product/1
  Trigonometric Function2/1 -> Trigonometric Function5/1
  Trigonometric Function5/1 -> eta/1, [eta]
  [V] -> Product/1, Product3/1
  [psi] -> Trigonometric Function3/1, Trigonometric Function4/1
  Trigonometric Function3/1 -> Product/2
  Trigonometric Function4/1 -> Product3/2
  Product3/1 -> Mux/1
  Product/1 -> Mux/2
  Constant/1 -> Mux/3
  Mux/1 -> Integrator2/1
  Integrator2/1 -> puav/1, [puav]
  Selector1/1 -> Dot Product/2, norm1/1(In1)
  norm2/1(Out1) -> [rho]
  [V] -> Product1/1
  Mux1/1 -> Scope1/1
  [eta] -> Trigonometric Function7/1
  Add1/1 -> Divide/1
  Gain1/1 -> Add1/1
  Trigonometric Function7/1 -> Saturation1/1
  Constant4/1 -> Divide/2
  Product6/1 -> Selector2/1
  [Laplacian] -> Product6/1
  lambda/1 -> Product6/2
  Divide/1 -> [Vcmd]
  Selector2/1 -> Gain1/1
  Selector3/1 -> Sum6/1
  Selector4/1 -> Sum6/2
  Trigonometric Function/1 -> MATLAB Function/2(lambda)
  Divide3/1 -> Trigonometric Function/1
  MATLAB Function/1(y) -> Derivative/1, Mux1/1, Integrator3/2, [lambda]
  Derivative/1 -> Rate Limiter/1
  Integrator3/1 -> Add2/1, Mux1/2, lamactual/1
  Add2/1 -> lam/1
  Constant8/1 -> Add2/2
  Sum/1 -> PID Controller1/1
  [Vcmd] -> Saturation2/1
  [psicmd] -> Sum3/1
  Sum3/1 -> [psi]
  [rho] -> Sum4/1
  Constant6/1 -> Sum4/2
  Sum4/1 -> roh_e/1, [rho_e]
  Saturation1/1 -> Divide/3
  Saturation/1 -> vel/1, [V], Sum/2, Mux4/1
  Integrator/1 -> Saturation/1
  PID Controller1/1 -> Integrator/1
  Mux4/1 -> Scope7/1
  Saturation2/1 -> Mux4/2, Integrator/2, Sum/1
